simulink model "AcousticNoiseCancellation"  (Simulink 6.5)
settings: Solver=FixedStepDiscrete  StartTime=0.0  StopTime=0.05  RelTol=1e-3
undefined symbols (not defined in the file or in its folder): get
libraries: simulink x1, dspadpt3 x1, dspsnks4 x1, dspsrcs4 x1
settings Model: Creator=Administrator  LastModifiedBy=Administrator

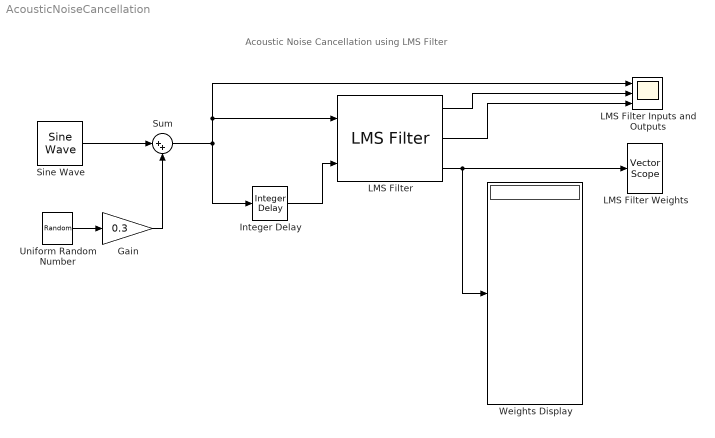
== system AcousticNoiseCancellation ==
  note: Acoustic Noise Cancellation using LMS Filter
  Gain : Gain  Gain=0.3
  Integer Delay : simulink/Discrete/Integer Delay  vinit=0.0  samptime=-1  NumDelays=50
  LMS Filter : dspadpt3/LMS Filter  DialogController=dspDDGCreate  DialogControllerArgs=DataTag0  Algo=LMS  L=12  stepflag=Dialog  mu=0.005  leakage=1  ic=0  Adapt=off  resetflag=None  weights=on  secondCoeffMode=User-defined  secondCoeffWordLength=2  secondCoeffFracLength=15  accum2Mode=User-defined  accum2FracLength=20  prodOutput2Mode=User-defined  prodOutput2FracLength=20  prodOutput3Mode=User-defined  prodOutput3FracLength=20  prodOutput4Mode=User-defined  prodOutput4FracLength=20  quotientMode=User-defined  quotientFracLength=20  roundingMode=Floor  overflowMode=off  addnparflag=off
  LMS Filter Inputs and Outputs : Scope  NumInputPorts=3
      settings: YMin=-2~-2~-2  YMax=2~2~2  SaveName=ScopeData3
  LMS Filter Weights : dspsnks4/Vector Scope  DialogController=dspdialog.VectorScope  DialogControllerArgs=DataTag1  ScopeProperties=on  Domain=Time  HorizSpan=12  DisplayProperties=off  AxisGrid=on  Memory=off  FrameNumber=on  AxisLegend=off  AxisZoom=off  OpenScopeAtSimStart=on  OpenScopeImmediately=off  FigPos=get(0,'defaultfigureposition')  AxisProperties=off  XUnits=Hertz  XRange=[0...Fs/2]  InheritXIncr=on  XIncr=1  XLabel=Time  YUnits=dB  YLabel=Amplitude  LineProperties=off
      settings: YMin=-0.3  YMax=0.3
  Sine Wave : dspsrcs4/Sine Wave  Amplitude=1  Frequency=200  Phase=0  SampleMode=Discrete  OutComplex=Real  CompMethod=Trigonometric fcn  TableSize=Speed  SampleTime=1/8000  SamplesPerFrame=1  dataType=double  wordLen=16  udDataType=sfix(16)  fracBitsMode=Best precision  numFracBits=15  ResetState=Restart at time zero
  Sum : Sum  Inputs=|++
  Uniform Random Number : UniformRandomNumber  SampleTime=0
  Weights Display : Display
  wires:
  Sine Wave/1 -> Sum/1
  Uniform Random Number/1 -> Gain/1
  Sum/1 -> Integer Delay/1, LMS Filter/1, LMS Filter Inputs and Outputs/1
  Integer Delay/1 -> LMS Filter/2
  LMS Filter/2 -> LMS Filter Inputs and Outputs/3
  LMS Filter/1 -> LMS Filter Inputs and Outputs/2
  LMS Filter/3 -> Weights Display/1, LMS Filter Weights/1
  Gain/1 -> Sum/2
